simulink model "testst"  (R2021a)
settings: Solver=VariableStepAuto  StartTime=0.0  StopTime=10  MaxStep=1  RelTol=1e-3
undefined symbols (not defined in the file or in its folder): DiscIntNeverNeededParam
libraries: vrlib x2, simulink x1
settings Model: Creator=Aero  LastModifiedBy=Aero

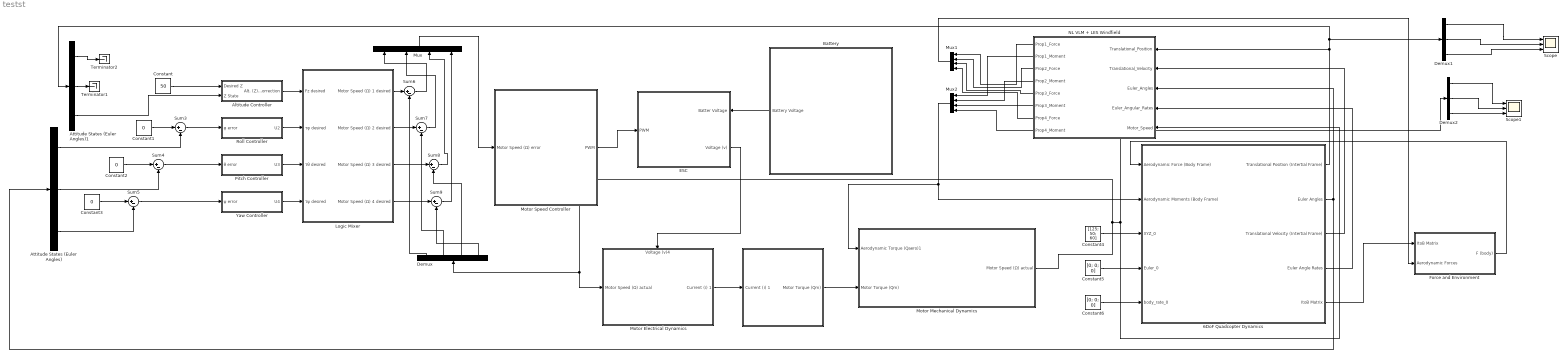
== system testst ==
  " " : Subsystem
  " Battery" : Subsystem
      settings: PortSchema="{\"entries\":[{\"content\":{\"sides\":[{\"content\":{\"connectorIds\":[\"Out1\"]},\"type\":\"ConnectorPlacement.EquallySpacedRectSide\",\"uuid\":\"23e9748a-abce-4ee5-9440-af4496418c11\"},{\"content\":{\"connectorIds\":[],\"side\":\"RIGHT\"},\"type\":\"ConnectorPlacement.EquallySpacedRectSide\",\"uuid\":\"b4057f8a-30b7-4429-a81e-64bcf25e7e2c\"},{\"content\":{\"connectorIds\":[],\"side\":\"TOP\"},\"type\":\"ConnectorPlacement.EquallySpacedRectSide\",\"uuid\":\"344446c6-3826-4594-b6bc-b6beed8e8252\"}]},\"type\":\"ConnectorPlacement.EquallySpacedConnector\",\"uuid\":\"0c8d6b35-4888-4c27-8968-32d9a485fb71\"}],\"packageUris\":[\"http://schema.mathworks.com/mf0/Connector/R2020b\"],\"version\":\"1.0\"}"
  " ESC" : Subsystem
      settings: PortSchema="{\"entries\":[{\"content\":{\"sides\":[{\"content\":{\"connectorIds\":[\"In1\"]},\"type\":\"ConnectorPlacement.EquallySpacedRectSide\",\"uuid\":\"2a15e5cd-7307-4c94-800f-101ac67c4ed6\"},{\"content\":{\"connectorIds\":[\"In2\",\"Out1\"],\"side\":\"RIGHT\"},\"type\":\"ConnectorPlacement.EquallySpacedRectSide\",\"uuid\":\"0f15f77e-bf35-4abe-b461-21a8655183cc\"},{\"content\":{\"connectorIds\":[],\"side\":\"TOP\"},\"type\":\"ConnectorPlacement.EquallySpacedRectSide\",\"uuid\":\"f61dcab0-36de-4d8e-9439-4c2551012467\"}]},\"type\":\"ConnectorPlacement.EquallySpacedConnector\",\"uuid\":\"9950464a-3a43-4c6a-9b16-9944baed22d9\"}],\"packageUris\":[\"http://schema.mathworks.com/mf0/Connector/R2020b\"],\"version\":\"1.0\"}"
  6DoF Quadcopter Dynamics : Subsystem
  Altitude Controller : Subsystem
  Attitude States (Euler Angles) : Demux  Outputs=3
  Attitude States (Euler Angles)1 : Demux  Outputs=3
  Constant : Constant  Value=50
  Constant1 : Constant  Value=0
  Constant2 : Constant  Value=0
  Constant3 : Constant  Value=0
  Constant4 : Constant  Value=[125; 50; 60]
  Constant5 : Constant  Value=[0; 0; 0]
  Constant6 : Constant  Value=[0; 0; 0]
  Demux : Demux
  Demux1 : Demux  Outputs=3
  Demux2 : Demux  Outputs=3
  Force and Environment : Subsystem
  Logic Mixer : Subsystem
  Motor Electrical Dynamics : Subsystem
      settings: PortSchema="{\"entries\":[{\"content\":{\"sides\":[{\"content\":{\"connectorIds\":[\"In1\"]},\"type\":\"ConnectorPlacement.EquallySpacedRectSide\",\"uuid\":\"f2031c02-0eca-4899-9e77-e180fcc093a7\"},{\"content\":{\"connectorIds\":[\"Out1\"],\"side\":\"RIGHT\"},\"type\":\"ConnectorPlacement.EquallySpacedRectSide\",\"uuid\":\"b34a3750-b9cf-412a-830e-44ef333463c8\"},{\"content\":{\"connectorIds\":[\"In2\"],\"side\":\"TOP\"},\"type\":\"ConnectorPlacement.EquallySpacedRectSide\",\"uuid\":\"69879be7-5af4-4622-a49e-5bb44b581c74\"}]},\"type\":\"ConnectorPlacement.EquallySpacedConnector\",\"uuid\":\"55dbe410-0e67-46f9-8761-f8d1e80fd108\"}],\"packageUris\":[\"http://schema.mathworks.com/mf0/Connector/R2020b\"],\"version\":\"1.0\"}"
  Motor Mechanical Dynamics : Subsystem
  Motor Speed Controller : Subsystem
  Mux : Mux
  Mux1 : Mux
  Mux2 : Mux
  "NL VLM + LES Windfield " : MATLAB Function  TreatAsAtomicUnit=on
  Pitch Controller : Subsystem
  Roll Controller : Subsystem
  Scope : Scope  NumInputPorts=3
  Scope1 : Scope  NumInputPorts=3
  Sum{3..9} (7 alike) : Sum  Inputs=|+-
  Terminator1 : Terminator
  Terminator2 : Terminator
  Yaw Controller : Subsystem
  wires:
  Motor Mechanical Dynamics/1(Motor Speed (Ω) actual) -> Demux2/1, "NL VLM + LES Windfield "/5(Motor_Speed), Demux/1, Motor Electrical Dynamics/1(Motor Speed (Ω) actual)
  6DoF Quadcopter Dynamics/1(Translational Position (Intertial Frame)) -> Attitude States (Euler Angles)1/1, Demux1/1, "NL VLM + LES Windfield "/1(Translational_Position)
  6DoF Quadcopter Dynamics/4(Euler Angle Rates) -> "NL VLM + LES Windfield "/4(Euler_Angular_Rates)
  6DoF Quadcopter Dynamics/3(Translational Velocity (Intertial Frame)) -> "NL VLM + LES Windfield "/2(Translational_Velocity)
  Roll Controller/1(U2) -> Logic Mixer/2(τφ desired)
  Pitch Controller/1(U3) -> Logic Mixer/3(τθ desired)
  Yaw Controller/1(U4) -> Logic Mixer/4(τψ desired)
  Constant/1 -> Altitude Controller/1(Desired Z)
  Sum3/1 -> Roll Controller/1(φ error)
  Sum4/1 -> Pitch Controller/1(θ error)
  Sum5/1 -> Yaw Controller/1(ψ error)
  Constant1/1 -> Sum3/1
  Constant2/1 -> Sum4/1
  Constant3/1 -> Sum5/1
  Attitude States (Euler Angles)/3 -> Sum5/2
  Attitude States (Euler Angles)/2 -> Sum4/2
  Attitude States (Euler Angles)/1 -> Sum3/2
  Altitude Controller/1(Alt. (Z) Correction) -> Logic Mixer/1(Fz desired)
  Constant4/1 -> 6DoF Quadcopter Dynamics/3(XYZ_0)
  Constant6/1 -> 6DoF Quadcopter Dynamics/5(body_rate_0)
  Constant5/1 -> 6DoF Quadcopter Dynamics/4(Euler_0)
  6DoF Quadcopter Dynamics/2(Euler Angles) -> Attitude States (Euler Angles)/1, "NL VLM + LES Windfield "/3(Euler_Angles)
  Attitude States (Euler Angles)1/3 -> Altitude Controller/2(Z State)
  Attitude States (Euler Angles)1/1 -> Terminator2/1
  Attitude States (Euler Angles)1/2 -> Terminator1/1
  Logic Mixer/2(Motor Speed (Ω) 2 desired) -> Sum7/1
  Logic Mixer/1(Motor Speed (Ω) 1 desired) -> Sum6/1
  Logic Mixer/3(Motor Speed (Ω) 3 desired) -> Sum8/1
  Logic Mixer/4(Motor Speed (Ω) 4 desired) -> Sum9/1
  Mux/1 -> Motor Speed Controller/1(Motor Speed (Ω) error)
  Sum6/1 -> Mux/1
  Sum7/1 -> Mux/2
  Sum8/1 -> Mux/3
  Sum9/1 -> Mux/4
  " Battery"/1(Battery Voltage) -> " ESC"/2(Batter Voltage)
  " ESC"/1(Voltage (v)) -> Motor Electrical Dynamics/2(Voltage (v)4)
  Motor Speed Controller/1(PWM) -> " ESC"/1("PWM ")
  " "/1(Motor Torque (Qm)) -> Motor Mechanical Dynamics/2(Motor Torque (Qm))
  Motor Electrical Dynamics/1(Current (i) 1) -> " "/1(Current (i) 1)
  6DoF Quadcopter Dynamics/5(ItoB Matrix) -> Force and Environment/1(ItoB Matrix)
  Force and Environment/1(F (body)) -> 6DoF Quadcopter Dynamics/1(Aerodynamic Force (Body Frame))
  Demux/1 -> Sum6/2
  Demux/2 -> Sum7/2
  Demux/3 -> Sum8/2
  Demux/4 -> Sum9/2
  "NL VLM + LES Windfield "/1(Prop1_Force) -> Mux1/1
  "NL VLM + LES Windfield "/5(Prop3_Force) -> Mux1/3
  "NL VLM + LES Windfield "/3(Prop2_Force) -> Mux1/2
  "NL VLM + LES Windfield "/7(Prop4_Force) -> Mux1/4
  "NL VLM + LES Windfield "/2(Prop1_Moment) -> Mux2/1
  "NL VLM + LES Windfield "/4(Prop2_Moment) -> Mux2/2
  "NL VLM + LES Windfield "/6(Prop3_Moment) -> Mux2/3
  "NL VLM + LES Windfield "/8(Prop4_Moment) -> Mux2/4
  Mux1/1 -> Force and Environment/2(Aerodynamic Forces)
  Mux2/1 -> Motor Mechanical Dynamics/1(Aerodynamic Torque (Qaero)1), 6DoF Quadcopter Dynamics/2(Aerodynamic Moments (Body Frame))
  Demux1/3 -> Scope/3
  Demux1/2 -> Scope/2
  Demux1/1 -> Scope/1
  Demux2/3 -> Scope1/3
  Demux2/2 -> Scope1/2
  Demux2/1 -> Scope1/1

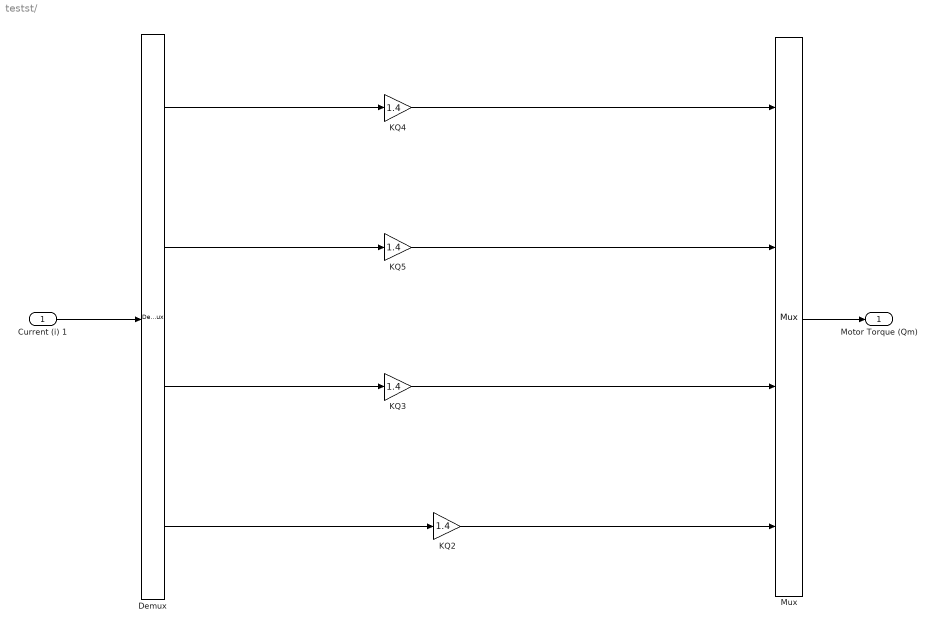
== system testst/  ==
  Current (i) 1 : Inport
  Demux : Demux
  KQ{2..5} (4 alike) : Gain  Gain=1.4
  Mux : Mux
  Motor Torque (Qm) : Outport
  wires:
  KQ2/1 -> Mux/4
  Demux/1 -> KQ4/1
  Demux/2 -> KQ5/1
  Demux/4 -> KQ2/1
  Demux/3 -> KQ3/1
  Current (i) 1/1 -> Demux/1
  Mux/1 -> Motor Torque (Qm)/1
  KQ3/1 -> Mux/3
  KQ5/1 -> Mux/2
  KQ4/1 -> Mux/1

== system testst/ Battery ==
  Constant : Constant  Value=300
  Battery Voltage : Outport
  wires:
  Constant/1 -> Battery Voltage/1

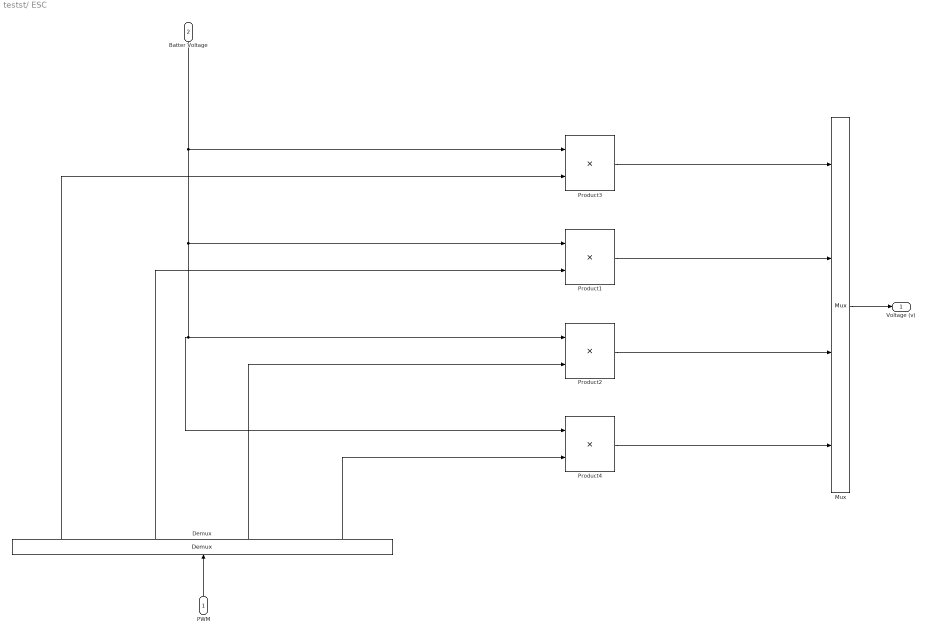
== system testst/ ESC ==
  "PWM " : Inport
  Batter Voltage : Inport  Port=2
  Demux : Demux
  Mux : Mux
  Product{1..4} (4 alike) : Product
  Voltage (v) : Outport
  wires:
  Demux/4 -> Product4/2
  Demux/3 -> Product2/2
  Product2/1 -> Mux/3
  Product1/1 -> Mux/2
  "PWM "/1 -> Demux/1
  Batter Voltage/1 -> Product4/1, Product2/1, Product1/1, Product3/1
  Product3/1 -> Mux/1
  Demux/1 -> Product3/2
  Product4/1 -> Mux/4
  Demux/2 -> Product1/2
  Mux/1 -> Voltage (v)/1

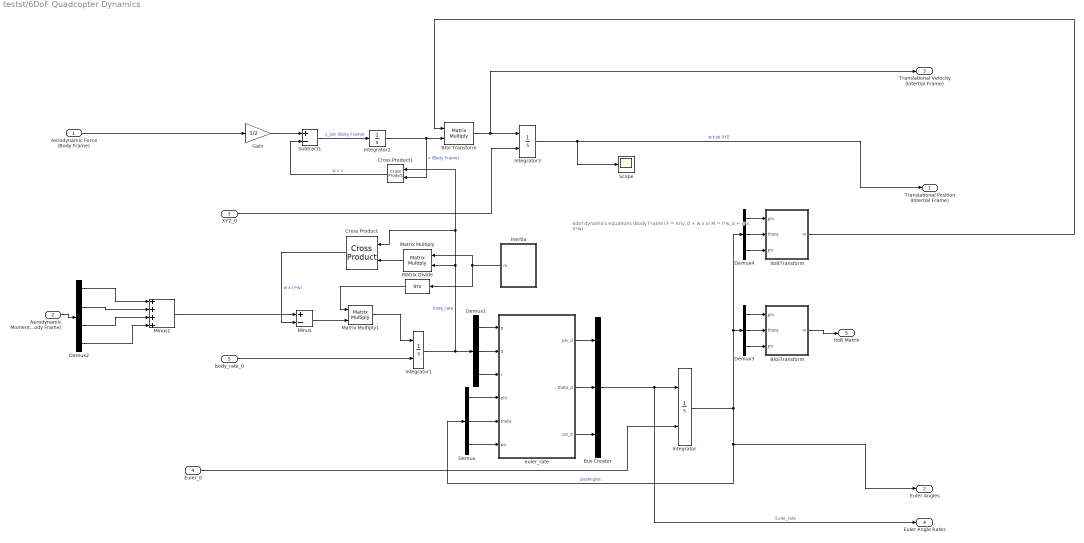
== system testst/6DoF Quadcopter Dynamics ==
  note: 6dof dynamics equations
      | (Body Frame)
      |
      | F = m(v_d + w x v)
      | M = I*w_d + w x (I*w)
  Aerodynamic Force (Body Frame) : Inport
  Aerodynamic Moments (Body Frame) : Inport  Port=2
  XYZ_0 : Inport  Port=3
  Euler_0 : Inport  Port=4
  body_rate_0 : Inport  Port=5
  BtoI Transform : Product  Multiplication=Matrix(*)
  BtoITransform : MATLAB Function  TreatAsAtomicUnit=on
  Bus Creator : BusCreator  Inputs=3
  Cross Product : vrlib/Utilities/Cross Product
  Cross Product1 : vrlib/Utilities/Cross Product
  Demux{,1,3..4} (4 alike) : Demux  Outputs=3
  Demux2 : Demux
  Gain : Gain  Gain=1/2
  Inertia : MATLAB Function  TreatAsAtomicUnit=on
  Integrator : Integrator  InitialConditionSource=external  ContinuousStateAttributes='EulerAngle'
  Integrator1 : Integrator  InitialConditionSource=external  ContinuousStateAttributes='EulerAngle'
  Integrator2 : Integrator
  Integrator3 : Integrator  InitialConditionSource=external
  ItoBTransform : MATLAB Function  TreatAsAtomicUnit=on
  Matrix Divide : Product  Inputs=/  Multiplication=Matrix(*)
  Matrix Multiply : Product  Multiplication=Matrix(*)
  Matrix Multiply1 : Product  Multiplication=Matrix(*)
  Minus : Sum  Inputs=+-
  Minus1 : Sum  Inputs=++++
  Scope : Scope
  Subtract1 : Sum  Inputs=+-
  euler_rate : MATLAB Function  TreatAsAtomicUnit=on
  Translational Position (Intertial Frame) : Outport
  Euler Angles : Outport  Port=2
  Translational Velocity (Intertial Frame) : Outport  Port=3
  Euler Angle Rates : Outport  Port=4
  ItoB Matrix : Outport  Port=5
  wires:
  Demux4/2 -> ItoBTransform/2(theta)
  euler_rate/1(phi_d) -> Bus Creator/1
  Bus Creator/1 -> Euler Angle Rates/1, Integrator/1  "Euler_rate"
  Matrix Multiply/1 -> Cross Product/2
  Inertia/1(m) -> Matrix Multiply/1, Matrix Divide/1
  Demux3/2 -> BtoITransform/2(theta)
  Demux/2 -> euler_rate/5(theta)
  Demux4/1 -> ItoBTransform/1(phi)
  Subtract1/1 -> Integrator2/1  "v_dot (Body Frame)"
  Cross Product1/1 -> Subtract1/2  "w x v"
  Demux1/1 -> euler_rate/1(p)
  Demux/3 -> euler_rate/6(psi)
  euler_rate/2(theta_d) -> Bus Creator/2
  Euler_0/1 -> Integrator/2
  Integrator3/1 -> Translational Position (Intertial Frame)/1, Scope/1  "actual XYZ"
  Cross Product/1 -> Minus/2  "w x (I*w)"
  body_rate_0/1 -> Integrator1/2
  Demux3/3 -> BtoITransform/3(psi)
  euler_rate/3(psi_d) -> Bus Creator/3
  Demux4/3 -> ItoBTransform/3(psi)
  Gain/1 -> Subtract1/1
  Demux3/1 -> BtoITransform/1(phi)
  Demux1/3 -> euler_rate/3(r)
  XYZ_0/1 -> Integrator3/2
  Integrator/1 -> Euler Angles/1, Demux/1, Demux4/1, Demux3/1  "ulerAngles"
  Demux/1 -> euler_rate/4(phi)
  Integrator2/1 -> BtoI Transform/2, Cross Product1/2  "v (Body Frame)"
  Integrator1/1 -> Cross Product1/1, Cross Product/1, Matrix Multiply/2, Demux1/1  "body_rate"
  Demux1/2 -> euler_rate/2(q)
  BtoI Transform/1 -> Translational Velocity (Intertial Frame)/1, Integrator3/1
  Minus/1 -> Matrix Multiply1/2
  Matrix Multiply1/1 -> Integrator1/1
  Matrix Divide/1 -> Matrix Multiply1/1
  BtoITransform/1(m) -> ItoB Matrix/1
  Aerodynamic Force (Body Frame)/1 -> Gain/1
  ItoBTransform/1(m) -> BtoI Transform/1
  Aerodynamic Moments (Body Frame)/1 -> Demux2/1
  Demux2/1 -> Minus1/1
  Demux2/2 -> Minus1/2
  Demux2/3 -> Minus1/3
  Demux2/4 -> Minus1/4
  Minus1/1 -> Minus/1

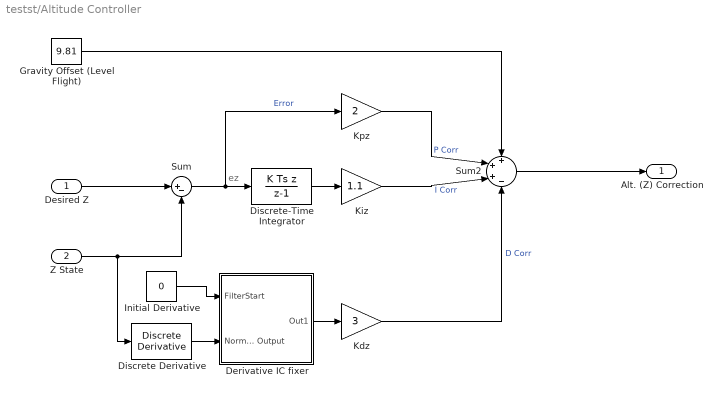
== system testst/Altitude Controller ==
  note: ez
  Desired Z : Inport
  Z State : Inport  Port=2
  Derivative IC fixer : Subsystem
  Discrete Derivative : simulink/Discrete/Discrete Derivative  gainval=1.0  ICPrevScaledInput=0.0  OutMin=[]  OutMax=[]  OutDataType=fixdt(1, 16)  OutScaling=2^-10  DoSatur=off
  Discrete-Time Integrator : DiscreteIntegrator  IntegratorMethod=Integration: Backward Euler  gainval=1.1  SampleTime=-1  LimitOutput=on  UpperSaturationLimit=1  LowerSaturationLimit=-1  ICPrevOutput=DiscIntNeverNeededParam  ICPrevScaledInput=DiscIntNeverNeededParam
  Gravity Offset (Level Flight) : Constant  Value=9.81
  Initial Derivative : Constant  Value=0
  Kdz : Gain  Gain=3
  Kiz : Gain  Gain=1.1
  Kpz : Gain  Gain=2
  Sum : Sum  Inputs=|+-
  Sum2 : Sum  Inputs=+++-
  Alt. (Z) Correction : Outport
  wires:
  Desired Z/1 -> Sum/1
  Sum/1 -> Discrete-Time Integrator/1, Kpz/1  "Error"
  Kdz/1 -> Sum2/4  "D Corr"
  Derivative IC fixer/1(Out1) -> Kdz/1
  Discrete Derivative/1 -> Derivative IC fixer/2(Normal Output)
  Kiz/1 -> Sum2/3  "I Corr"
  Kpz/1 -> Sum2/2  "P Corr"
  Discrete-Time Integrator/1 -> Kiz/1
  Initial Derivative/1 -> Derivative IC fixer/1(FilterStart)
  Z State/1 -> Discrete Derivative/1, Sum/2
  Sum2/1 -> Alt. (Z) Correction/1
  Gravity Offset (Level Flight)/1 -> Sum2/1

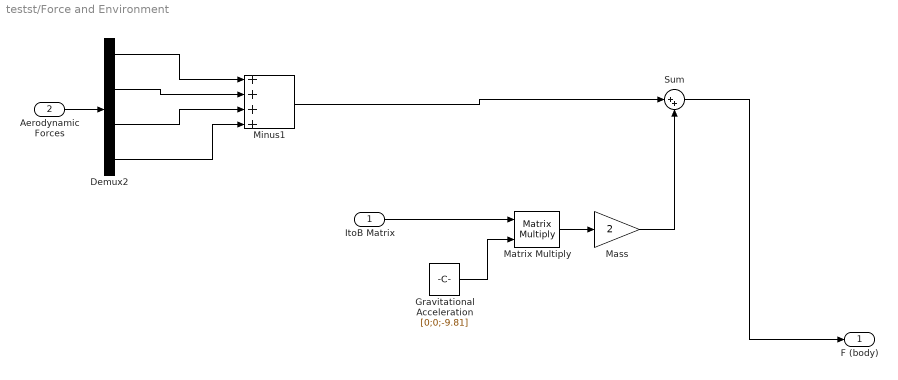
== system testst/Force and Environment ==
  ItoB Matrix : Inport
  Aerodynamic Forces : Inport  Port=2
  Demux2 : Demux
  Gravitational Acceleration : Constant  Value=[0;0;-9.81]  SampleTime=0.01
  Mass : Gain  Gain=2
  Matrix Multiply : Product  Multiplication=Matrix(*)
  Minus1 : Sum  Inputs=++++
  Sum : Sum  Inputs=|++
  F (body) : Outport
  wires:
  Gravitational Acceleration/1 -> Matrix Multiply/2
  ItoB Matrix/1 -> Matrix Multiply/1
  Matrix Multiply/1 -> Mass/1
  Sum/1 -> F (body)/1
  Mass/1 -> Sum/2
  Aerodynamic Forces/1 -> Demux2/1
  Demux2/4 -> Minus1/4
  Demux2/3 -> Minus1/3
  Demux2/2 -> Minus1/2
  Demux2/1 -> Minus1/1
  Minus1/1 -> Sum/1

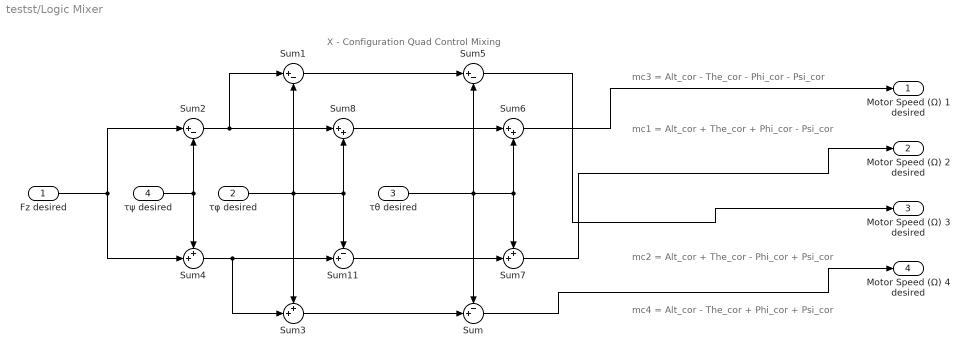
== system testst/Logic Mixer ==
  note: X - Configuration Quad Control Mixing
  note: mc3 = Alt_cor - The_cor - Phi_cor - Psi_cor
  note: mc2 = Alt_cor + The_cor - Phi_cor + Psi_cor
  note: mc1 = Alt_cor + The_cor + Phi_cor - Psi_cor
  note: mc4 = Alt_cor - The_cor + Phi_cor + Psi_cor
  Fz desired : Inport
  τφ desired : Inport  Port=2
  τθ desired : Inport  Port=3
  τψ desired : Inport  Port=4
  Sum : Sum  Inputs=-+|
  Sum1 : Sum  Inputs=|+-
  Sum11 : Sum  Inputs=-+|
  Sum2 : Sum  Inputs=|+-
  Sum3 : Sum  Inputs=++|
  Sum4 : Sum  Inputs=++|
  Sum5 : Sum  Inputs=|+-
  Sum6 : Sum  Inputs=|++
  Sum7 : Sum  Inputs=++|
  Sum8 : Sum  Inputs=|++
  Motor Speed (Ω) 1 desired : Outport
  Motor Speed (Ω) 2 desired : Outport  Port=2
  Motor Speed (Ω) 3 desired : Outport  Port=3
  Motor Speed (Ω) 4 desired : Outport  Port=4
  wires:
  Sum11/1 -> Sum7/2
  τθ desired/1 -> Sum7/1, Sum6/2, Sum5/2, Sum/1
  Sum8/1 -> Sum6/1
  Sum6/1 -> Motor Speed (Ω) 1 desired/1
  Sum7/1 -> Motor Speed (Ω) 2 desired/1
  τψ desired/1 -> Sum4/1, Sum2/2
  Sum2/1 -> Sum8/1, Sum1/1
  Sum4/1 -> Sum3/2, Sum11/2
  Sum1/1 -> Sum5/1
  τφ desired/1 -> Sum3/1, Sum1/2, Sum8/2, Sum11/1
  Sum3/1 -> Sum/2
  Fz desired/1 -> Sum2/1, Sum4/2
  Sum/1 -> Motor Speed (Ω) 4 desired/1
  Sum5/1 -> Motor Speed (Ω) 3 desired/1

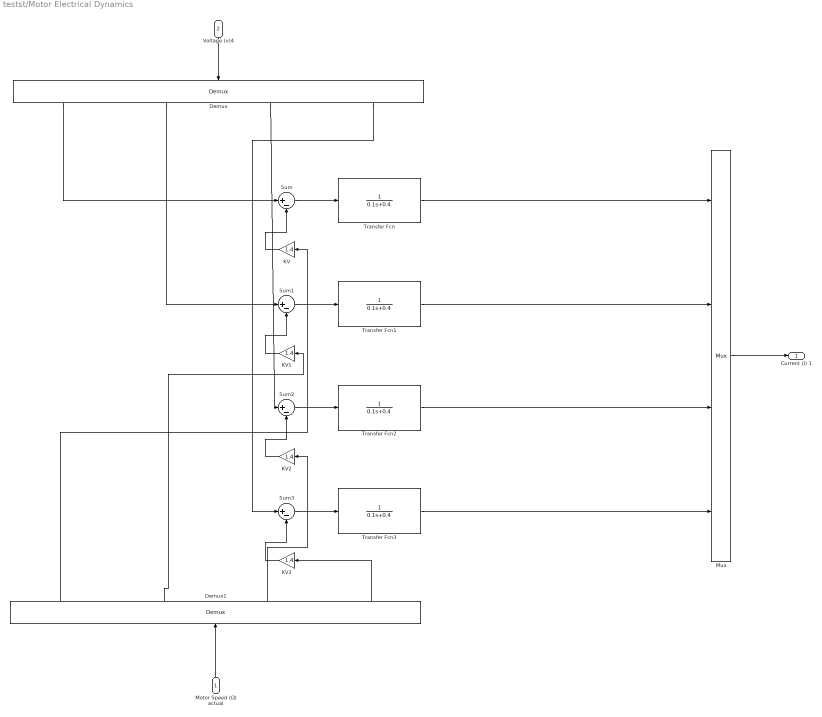
== system testst/Motor Electrical Dynamics ==
  Motor Speed (Ω) actual : Inport
  Voltage (v)4 : Inport  Port=2
  Demux : Demux
  Demux1 : Demux
  KV{,1..3} (4 alike) : Gain  Gain=1.4
  Mux : Mux
  Sum{,1..3} (4 alike) : Sum  Inputs=|+-
  Transfer Fcn{,1..3} (4 alike) : TransferFcn  Denominator=[0.1 0.4]
  Current (i) 1 : Outport
  wires:
  Transfer Fcn/1 -> Mux/1
  Demux/1 -> Sum/1
  Sum/1 -> Transfer Fcn/1
  KV/1 -> Sum/2
  Mux/1 -> Current (i) 1/1
  Demux1/1 -> KV/1
  Transfer Fcn1/1 -> Mux/2
  Demux/2 -> Sum1/1
  Sum1/1 -> Transfer Fcn1/1
  KV1/1 -> Sum1/2
  Transfer Fcn2/1 -> Mux/3
  Demux/3 -> Sum2/1
  Sum2/1 -> Transfer Fcn2/1
  KV2/1 -> Sum2/2
  Transfer Fcn3/1 -> Mux/4
  Demux/4 -> Sum3/1
  Sum3/1 -> Transfer Fcn3/1
  KV3/1 -> Sum3/2
  Demux1/2 -> KV1/1
  Demux1/3 -> KV2/1
  Demux1/4 -> KV3/1
  Motor Speed (Ω) actual/1 -> Demux1/1
  Voltage (v)4/1 -> Demux/1

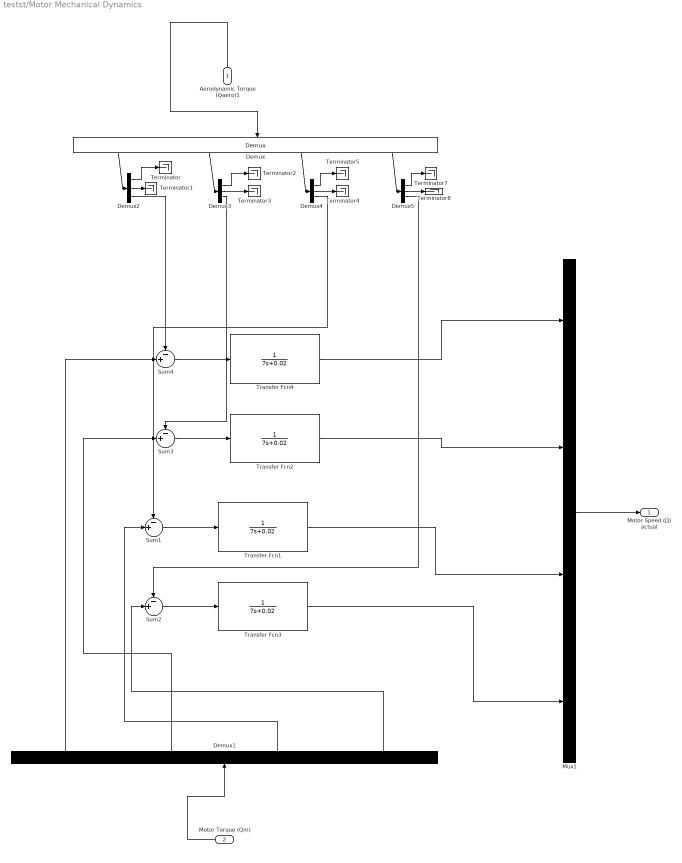
== system testst/Motor Mechanical Dynamics ==
  Aerodynamic Torque (Qaero)1 : Inport
  Motor Torque (Qm) : Inport  Port=2
  Demux : Demux
  Demux1 : Demux
  Demux{2..5} (4 alike) : Demux  Outputs=3
  Mux1 : Mux
  Sum{1..4} (4 alike) : Sum  Inputs=-+|
  Terminator{,1..5,7..8} (8 alike) : Terminator
  Transfer Fcn{1..4} (4 alike) : TransferFcn  Denominator=[7 0.02]
  Motor Speed (Ω) actual : Outport
  wires:
  Sum3/1 -> Transfer Fcn2/1
  Motor Torque (Qm)/1 -> Demux1/1
  Aerodynamic Torque (Qaero)1/1 -> Demux/1
  Sum1/1 -> Transfer Fcn1/1
  Sum2/1 -> Transfer Fcn3/1
  Sum4/1 -> Transfer Fcn4/1
  Demux1/4 -> Sum2/2
  Demux1/3 -> Sum1/2
  Demux1/2 -> Sum3/2
  Demux1/1 -> Sum4/2
  Mux1/1 -> Motor Speed (Ω) actual/1
  Transfer Fcn4/1 -> Mux1/1
  Transfer Fcn2/1 -> Mux1/2
  Transfer Fcn1/1 -> Mux1/3
  Transfer Fcn3/1 -> Mux1/4
  Demux/1 -> Demux2/1
  Demux2/3 -> Sum4/1
  Demux/2 -> Demux3/1
  Demux/3 -> Demux4/1
  Demux/4 -> Demux5/1
  Demux3/3 -> Sum3/1
  Demux4/3 -> Sum1/1
  Demux5/3 -> Sum2/1
  Demux2/1 -> Terminator/1
  Demux2/2 -> Terminator1/1
  Demux3/1 -> Terminator2/1
  Demux3/2 -> Terminator3/1
  Demux5/1 -> Terminator7/1
  Demux5/2 -> Terminator8/1
  Demux4/1 -> Terminator5/1
  Demux4/2 -> Terminator4/1

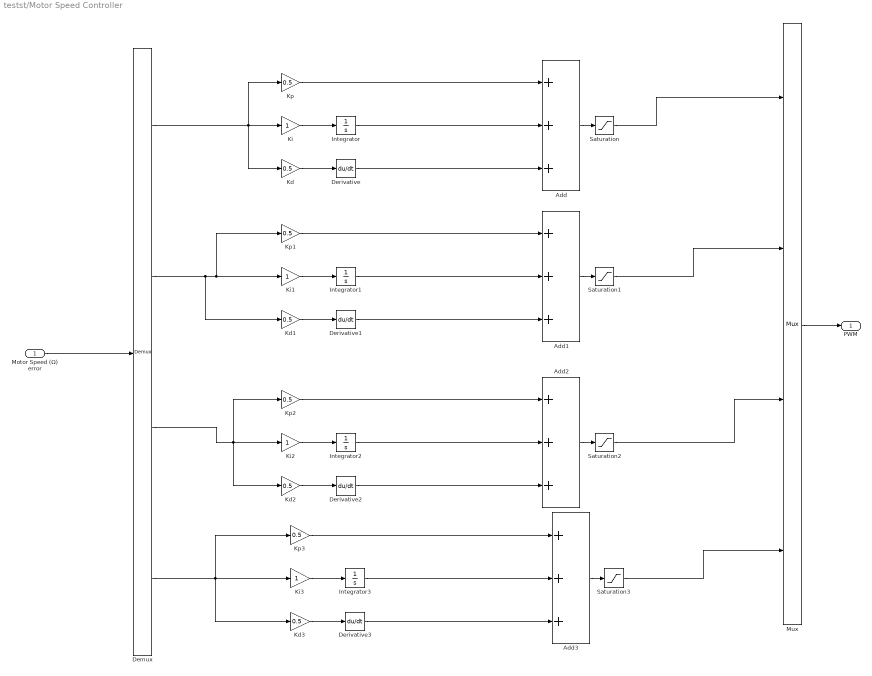
== system testst/Motor Speed Controller ==
  Motor Speed (Ω) error : Inport
  Add{,1..3} (4 alike) : Sum  Inputs=+++
  Demux : Demux
  Derivative{,1..3} (4 alike) : Derivative
  Integrator{,1..3} (4 alike) : Integrator
  Kd{,1..3} (4 alike) : Gain  Gain=0.5
  Ki{,1..3} (4 alike) : Gain
  Kp{,1..3} (4 alike) : Gain  Gain=0.5
  Mux : Mux
  Saturation{,1..3} (4 alike) : Saturate  UpperLimit=1  LowerLimit=0
  PWM : Outport
  wires:
  Kd/1 -> Derivative/1
  Derivative/1 -> Add/3
  Integrator/1 -> Add/2
  Ki/1 -> Integrator/1
  Kp/1 -> Add/1
  Add/1 -> Saturation/1
  Saturation/1 -> Mux/1
  Motor Speed (Ω) error/1 -> Demux/1
  Ki1/1 -> Integrator1/1
  Kp1/1 -> Add1/1
  Integrator1/1 -> Add1/2
  Add1/1 -> Saturation1/1
  Saturation1/1 -> Mux/2
  Kd1/1 -> Derivative1/1
  Derivative1/1 -> Add1/3
  Ki2/1 -> Integrator2/1
  Kp2/1 -> Add2/1
  Integrator2/1 -> Add2/2
  Add2/1 -> Saturation2/1
  Saturation2/1 -> Mux/3
  Kd2/1 -> Derivative2/1
  Derivative2/1 -> Add2/3
  Ki3/1 -> Integrator3/1
  Saturation3/1 -> Mux/4
  Derivative3/1 -> Add3/3
  Add3/1 -> Saturation3/1
  Integrator3/1 -> Add3/2
  Kd3/1 -> Derivative3/1
  Kp3/1 -> Add3/1
  Demux/1 -> Kd/1, Kp/1, Ki/1
  Demux/2 -> Kd1/1, Ki1/1, Kp1/1
  Demux/3 -> Kd2/1, Kp2/1, Ki2/1
  Demux/4 -> Kd3/1, Kp3/1, Ki3/1
  Mux/1 -> PWM/1

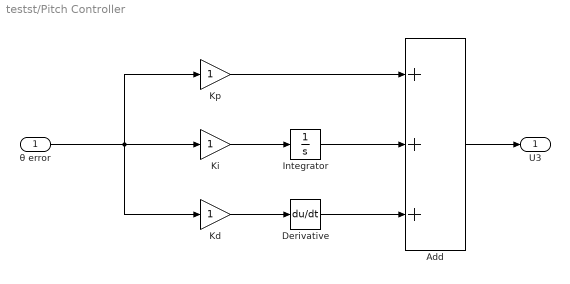
== system testst/Pitch Controller ==
  θ error : Inport
  Add : Sum  Inputs=+++
  Derivative : Derivative
  Integrator : Integrator
  Kd : Gain
  Ki : Gain
  Kp : Gain
  U3 : Outport
  wires:
  Add/1 -> U3/1
  θ error/1 -> Kd/1, Kp/1, Ki/1
  Kp/1 -> Add/1
  Integrator/1 -> Add/2
  Derivative/1 -> Add/3
  Kd/1 -> Derivative/1
  Ki/1 -> Integrator/1

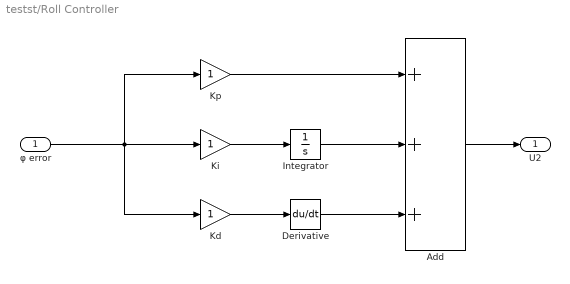
== system testst/Roll Controller ==
  φ error : Inport
  Add : Sum  Inputs=+++
  Derivative : Derivative
  Integrator : Integrator
  Kd : Gain
  Ki : Gain
  Kp : Gain
  U2 : Outport
  wires:
  Derivative/1 -> Add/3
  Add/1 -> U2/1
  φ error/1 -> Kd/1, Kp/1, Ki/1
  Integrator/1 -> Add/2
  Kp/1 -> Add/1
  Ki/1 -> Integrator/1
  Kd/1 -> Derivative/1

== system testst/Yaw Controller ==
  ψ error : Inport
  Add : Sum  Inputs=+++
  Derivative : Derivative
  Integrator : Integrator
  Kd : Gain
  Ki : Gain
  Kp : Gain
  U4 : Outport
  wires:
  Ki/1 -> Integrator/1
  Kd/1 -> Derivative/1
  ψ error/1 -> Kd/1, Kp/1, Ki/1
  Add/1 -> U4/1
  Kp/1 -> Add/1
  Integrator/1 -> Add/2
  Derivative/1 -> Add/3

== system testst/Altitude Controller/Derivative IC fixer ==
  FilterStart : Inport
  Normal Output : Inport  Port=2
  Constant : Constant
  IC : InitialCondition  Value=0
  Switch : Switch  Criteria=u2 ~= 0
  Out1 : Outport
  wires:
  Switch/1 -> Out1/1
  FilterStart/1 -> Switch/3
  IC/1 -> Switch/2
  Constant/1 -> IC/1
  Normal Output/1 -> Switch/1

== matlab function testst/6DoF Quadcopter Dynamics/BtoITransform ==
  data: phi input; m output; theta input; psi input
function m = fcn(phi,theta,psi)
    T_BtoV2 = [[1 0 0];[0 cos(-phi) sin(-phi)];[0 -sin(-phi) cos(-phi)]];
    T_V2toV1 = [[cos(-theta) 0 -sin(-theta)];[0 1 0];[sin(-theta) 0 cos(-theta)]];
    T_V1toI = [[cos(-psi) sin(-psi) 0];[-sin(-psi) cos(-psi) 0];[0 0 1]];
    m = T_V1toI*T_V2toV1*T_BtoV2;

== matlab function testst/6DoF Quadcopter Dynamics/euler_rate ==
  data: p input; phi_d output; q input; r input; phi input; theta input; theta_d output; psi_d output; psi input
function [phi_d,theta_d,psi_d] = fcn(p,q,r,phi,theta,psi)
    D = [[1 sin(phi)*tan(theta) cos(phi)*tan(theta)];
         [0 cos(phi) -sin(phi)];
         [0 sin(phi)/cos(theta) cos(phi)/cos(theta)]];
    euler_rate = D*[p;q;r]
    phi_d = euler_rate(1)
    theta_d = euler_rate(2)
    psi_d = euler_rate(3)

== matlab function testst/6DoF Quadcopter Dynamics/Inertia ==
  data: m output
function m =    Inertia

        m =  [[0.0045 0 0];[0 0.0045 0];[0 0 0.009]];

== matlab function testst/NL VLM + LES Windfield  ==
  data: Translational_Position input; Prop1_Force output; Translational_Velocity input; Euler_Angles input; Euler_Angular_Rates input; Motor_Speed input; Prop1_Moment output; Prop2_Force output; Prop2_Moment output; Prop3_Force output; Prop3_Moment output; Prop4_Force output; Prop4_Moment output
function [Prop1_Force, Prop1_Moment, Prop2_Force, Prop2_Moment, Prop3_Force, Prop3_Moment, Prop4_Force, Prop4_Moment] = Python_Aerodynamics(Translational_Position, Translational_Velocity, Euler_Angles, Euler_Angular_Rates, Motor_Speed)
    % Call the external function to get individual propeller forces and moments
    [prop1_force, prop1_moment, prop2_force, prop2_moment, prop3_force, prop3_moment, prop4_force, prop4_moment] = callPythonAerodynamics(Translational_Position, Translational_Velocity, Euler_Angles, Euler_Angular_Rates, Motor_Speed);
    
    % Output each propeller's force and moment as separate signals
    Prop1_Force = prop1_force;  % 3x1 vector for propeller 1 force
    Prop1_Moment = prop1_moment;  % 3x1 vector for propeller 1 moment
    Prop2_Force = prop2_force;  % 3x1 vector for propeller 2 force
    Prop2_Moment = prop2_moment;  % 3x1 vector for propeller 2 moment
    Prop3_Force = prop3_force;  % 3x1 vector for propeller 3 force
    Prop3_Moment = prop3_moment;  % 3x1 vector for propeller 3 moment
    Prop4_Force = prop4_force;  % 3x1 vector for propeller 4 force
    Prop4_Moment = prop4_moment;  % 3x1 vector for propeller 4 moment
end

== matlab function testst/6DoF Quadcopter Dynamics/ItoBTransform ==
  data: phi input; m output; theta input; psi input
function m = fcn(phi,theta,psi)
    T_ItoV1 = [[cos(psi) sin(psi) 0];[-sin(psi) cos(psi) 0];[0 0 1]]; 
    T_V1toV2 = [[cos(theta) 0 -sin(theta)];[0 1 0];[sin(theta) 0 cos(theta)]];
    T_V2toB = [[1 0 0];[0 cos(phi) sin(phi)];[0 -sin(phi) cos(phi)]];
    m = T_V2toB*T_V1toV2*T_ItoV1
